simulink model "LinLongNormal_Aquila_ClawsGainSchedule_Discrete"  (Simulink 8.9)
settings: Solver=VariableStepAuto  StartTime=0.0  StopTime=50  RelTol=1e-3  EnableMultiTasking=on
PreLoadFcn:
  | AquilaDiscreteClawsParameters_GS
  | AquilaDiscreteModelParameters
model workspace: external: MAT-File (data not in the file)
undefined symbols (not defined in the file): AP_AltLoop_AltCmdLPFDenTau, AP_AltLoop_Kd0, AP_AltLoop_Ki0, AP_AltLoop_Ki_WindupMaxLim, AP_AltLoop_Ki_WindupMinLim, AP_AltLoop_Kp0, AP_ClimbRate_LPFDenTau, AP_ClimbRateLoop_ClimbRateCmdLPFDenTau, AP_ClimbRateLoop_Ki0, AP_ClimbRateLoop_Kp0, AP_ClimbRateLoop_LLFiltDenCoe0, AP_ClimbRateLoop_LLFiltNumCoe0, AP_ClimbRateLoop_MaxPitchCmdrad, AP_ClimbRateLoop_MinPitchCmdrad, AP_GndTrkLoop_CmdLPFDenTau, AP_GndTrkLoop_Kd0, AP_GndTrkLoop_Kp0, AP_GndTrkLoop_phiCmdMaxLimDeg, AP_GndTrkLoop_phiCmdMinLimDeg, AP_GndTrkLoop_phiRateCmdMaxLimDps, AP_GndTrkLoop_phiRateCmdMinLimDps, AP_PitchLoop_DerivLPFDenTau, AP_PitchLoop_Kd, AP_PitchLoop_Kff, AP_PitchLoop_Ki0, AP_PitchLoop_Kp0, AP_PitchLoop_Kq0, AP_PitchLoop_Notch1BWfactor, AP_PitchLoop_Notch1CosFreqNorm, AP_PitchLoop_qFdbkLFLLFiltDenCoe0, AP_PitchLoop_qFdbkLFLLFiltNumCoe0, AP_PitchLoop_qFdbkLLFiltDenCoe0, AP_PitchLoop_qFdbkLLFiltNumCoe0, AP_PitchLoop_thetaCmdLPFDenTau, AP_PitchLoop_wn_ElvRollOff, AP_PitchLoop_zeta_ElvRollOff, AP_PwrLoop_ClimbRateCmdLPFDenTau, AP_PwrLoop_Ki0, AP_PwrLoop_Kp0, AP_PwrLoop_Kvadv0, AP_PwrLoop_LLFiltDenCoe0, AP_PwrLoop_LLFiltNumCoe0, AP_PwrLoop_MaxThrCmdNorm, AP_PwrLoop_MinThrCmdNorm, AP_PwrLoop_wn_ThrRollOff, AP_PwrLoop_zeta_ThrRollOff, AP_RollLoop_ailCmdMaxLim, AP_RollLoop_ailCmdMinLim, AP_RollLoop_AilWindupMaxLim, AP_RollLoop_AilWindupMinLim, AP_RollLoop_Ki0, AP_RollLoop_Kp0, AP_RollLoop_KrollrateAdv0, AP_RollLoop_Notch1BWfactor, AP_RollLoop_Notch1CosFreqNorm, AP_RollLoop_pFdbkLFLLFiltDenCoe0, AP_RollLoop_pFdbkLFLLFiltNumCoe0, AP_RollLoop_pFdbkLLFiltDenCoe0, AP_RollLoop_pFdbkLLFiltNumCoe0, AP_RollLoop_phiErrLPFDenTau ... (+41)
libraries: discretizing x16, aerolibconvert2 x12, simulink x8
(part 2 of 2)

== system LinLongNormal_Aquila_ClawsGainSchedule_Discrete/Lateral_Directional_Control_Laws/RollLoop/Notch Filter 1 ==
  note: One of ways to implement it for the scheduling of the AP_RollLoop_Notch1CosFreqNorm across the flight envelop
  note: 2nd order IIR Notch filter
  u : Inport
  AP_RollLoop_Notch1BWfactor : Gain  Gain=AP_RollLoop_Notch1BWfactor
  AP_RollLoop_Notch1BWfactor1 : Gain  Gain=AP_RollLoop_Notch1BWfactor
  AP_RollLoop_Notch1BWfactor2 : Gain  Gain=AP_RollLoop_Notch1BWfactor
  AP_RollLoop_Notch1CosFreqNorm : Gain  Gain=AP_RollLoop_Notch1CosFreqNorm
  AP_RollLoop_Notch1CosFreqNorm1 : Gain  Gain=AP_RollLoop_Notch1CosFreqNorm
  Delay : Delay  DelayLength=1  InitialCondition=0  SampleTime=Ts
  Delay1 : Delay  DelayLength=1  InitialCondition=0  SampleTime=Ts
  Delay2 : Delay  InitialCondition=0  SampleTime=Ts
  Delay3 : Delay  InitialCondition=0  SampleTime=Ts
  Gain1 : Gain  Gain=-2
  Gain2 : Gain  Gain=0.4697
  Gain4 : Gain  Gain=2
  Gain5 : Gain  Gain=-1
  Sum : Sum  Inputs=|++
  Sum1 : Sum  Inputs=|++
  Sum2 : Sum  Inputs=|++
  Sum3 : Sum  Inputs=+++||
  y : Outport
  wires:
  Sum/1 -> Gain2/1
  AP_RollLoop_Notch1BWfactor/1 -> Sum/1
  AP_RollLoop_Notch1CosFreqNorm/1 -> Sum3/2
  u/1 -> Delay/1, Sum3/1, Delay2/1
  Sum1/1 -> y/1, Delay1/1, Delay3/1
  AP_RollLoop_Notch1BWfactor2/1 -> Gain5/1
  Delay3/1 -> AP_RollLoop_Notch1BWfactor2/1
  Gain1/1 -> AP_RollLoop_Notch1CosFreqNorm/1
  Delay1/1 -> AP_RollLoop_Notch1CosFreqNorm1/1
  Delay2/1 -> Sum3/3
  Delay/1 -> Gain1/1
  AP_RollLoop_Notch1CosFreqNorm1/1 -> Gain4/1
  Sum3/1 -> Sum/2, AP_RollLoop_Notch1BWfactor/1
  Gain2/1 -> Sum1/1
  Gain4/1 -> Sum2/2
  Gain5/1 -> Sum2/1
  AP_RollLoop_Notch1BWfactor1/1 -> Sum1/2
  Sum2/1 -> AP_RollLoop_Notch1BWfactor1/1

== system LinLongNormal_Aquila_ClawsGainSchedule_Discrete/Lateral_Directional_Control_Laws/RollLoop/Subsystem ==
  note: Return to the previous filter implementation for the opt script
  u : Inport
  pres_alt_m : Inport  Port=2
  DynPres : Inport  Port=3
  AP_RollLoop_pFdbkLLFiltDenCoe : Interpolation_n-D  Table=AP_RollLoop_pFdbkLLFiltDenCoe0  ExtrapMethod=Clip  InternalRulePriority=Speed
  AP_RollLoop_pFdbkLLFiltNumCoe : Interpolation_n-D  Table=AP_RollLoop_pFdbkLLFiltNumCoe0  ExtrapMethod=Clip  InternalRulePriority=Speed
  Delay : Delay  DelayLength=1  InitialCondition=0  SampleTime=Ts
  Prelookup1 : PreLookup  BreakpointsData=0:1500:12000  ExtrapMethod=Linear
  Prelookup2 : PreLookup  BreakpointsData=45:15:150  ExtrapMethod=Linear
  Product1 : Product
  Product2 : Product
  Sum : Sum  Inputs=|++
  Sum1 : Sum  Inputs=+|-
  y : Outport
  wires:
  DynPres/1 -> Prelookup2/1
  AP_RollLoop_pFdbkLLFiltNumCoe/1 -> Product1/2
  AP_RollLoop_pFdbkLLFiltDenCoe/1 -> Product2/2
  pres_alt_m/1 -> Prelookup1/1
  Prelookup1/1 -> AP_RollLoop_pFdbkLLFiltDenCoe/1, AP_RollLoop_pFdbkLLFiltNumCoe/1
  Prelookup1/2 -> AP_RollLoop_pFdbkLLFiltDenCoe/2, AP_RollLoop_pFdbkLLFiltNumCoe/2
  Prelookup2/1 -> AP_RollLoop_pFdbkLLFiltNumCoe/3, AP_RollLoop_pFdbkLLFiltDenCoe/3
  Prelookup2/2 -> AP_RollLoop_pFdbkLLFiltNumCoe/4, AP_RollLoop_pFdbkLLFiltDenCoe/4
  Sum/1 -> y/1, Product2/1
  u/1 -> Sum/1, Product1/1
  Sum1/1 -> Delay/1
  Product1/1 -> Sum1/1
  Delay/1 -> Sum/2
  Product2/1 -> Sum1/2

== system LinLongNormal_Aquila_ClawsGainSchedule_Discrete/Lateral_Directional_Control_Laws/RollLoop/Subsystem3 ==
  u : Inport
  AP_RollLoop_rollAdvLLFiltDenCoe : Gain  Gain=AP_RollLoop_rollAdvLLFiltDenCoe
  AP_RollLoop_rollAdvLLFiltNumCoe : Gain  Gain=AP_RollLoop_rollAdvLLFiltNumCoe
  Delay : Delay  DelayLength=1  InitialCondition=0  SampleTime=Ts
  Delay1 : Delay  DelayLength=1  InitialCondition=0  SampleTime=Ts
  Sum3 : Sum  Inputs=+|+|-
  y : Outport
  wires:
  AP_RollLoop_rollAdvLLFiltDenCoe/1 -> Sum3/3
  u/1 -> AP_RollLoop_rollAdvLLFiltNumCoe/1, Sum3/1
  Delay1/1 -> AP_RollLoop_rollAdvLLFiltDenCoe/1
  AP_RollLoop_rollAdvLLFiltNumCoe/1 -> Delay/1
  Delay/1 -> Sum3/2
  Sum3/1 -> y/1, Delay1/1

== system LinLongNormal_Aquila_ClawsGainSchedule_Discrete/Lateral_Directional_Control_Laws/RollLoop/Subsystem4 ==
  u : Inport
  pres_alt_m : Inport  Port=2
  DynPres : Inport  Port=3
  AP_RollLoop_pFdbkLFLLFiltDenCoe : Interpolation_n-D  Table=AP_RollLoop_pFdbkLFLLFiltDenCoe0  ExtrapMethod=Clip  InternalRulePriority=Speed
  AP_RollLoop_pFdbkLFLLFiltNumCoe : Interpolation_n-D  Table=AP_RollLoop_pFdbkLFLLFiltNumCoe0  ExtrapMethod=Clip  InternalRulePriority=Speed
  Delay : Delay  DelayLength=1  InitialCondition=0  SampleTime=Ts
  Prelookup1 : PreLookup  BreakpointsData=0:1500:12000  ExtrapMethod=Linear
  Prelookup2 : PreLookup  BreakpointsData=45:15:150  ExtrapMethod=Linear
  Product1 : Product
  Product2 : Product
  Sum : Sum  Inputs=|++
  Sum1 : Sum  Inputs=+|-
  y : Outport
  wires:
  DynPres/1 -> Prelookup2/1
  AP_RollLoop_pFdbkLFLLFiltNumCoe/1 -> Product1/2
  AP_RollLoop_pFdbkLFLLFiltDenCoe/1 -> Product2/2
  pres_alt_m/1 -> Prelookup1/1
  Prelookup1/1 -> AP_RollLoop_pFdbkLFLLFiltDenCoe/1, AP_RollLoop_pFdbkLFLLFiltNumCoe/1
  Prelookup1/2 -> AP_RollLoop_pFdbkLFLLFiltDenCoe/2, AP_RollLoop_pFdbkLFLLFiltNumCoe/2
  Prelookup2/1 -> AP_RollLoop_pFdbkLFLLFiltNumCoe/3, AP_RollLoop_pFdbkLFLLFiltDenCoe/3
  Prelookup2/2 -> AP_RollLoop_pFdbkLFLLFiltNumCoe/4, AP_RollLoop_pFdbkLFLLFiltDenCoe/4
  Sum/1 -> y/1, Product2/1
  u/1 -> Sum/1, Product1/1
  Sum1/1 -> Delay/1
  Product1/1 -> Sum1/1
  Delay/1 -> Sum/2
  Product2/1 -> Sum1/2

== system LinLongNormal_Aquila_ClawsGainSchedule_Discrete/Lateral_Directional_Control_Laws/YawLoop/Subsystem1 ==
  u : Inport
  pres_alt_m : Inport  Port=2
  DynPres : Inport  Port=3
  AP_YawRateLoop_LLFiltDenCoe : Interpolation_n-D  Table=AP_YawRateLoop_LLFiltDenCoe0  ExtrapMethod=Clip  InternalRulePriority=Speed
  AP_YawRateLoop_LLFiltNumCoe : Interpolation_n-D  Table=AP_YawRateLoop_LLFiltNumCoe0  ExtrapMethod=Clip  InternalRulePriority=Speed
  Delay : Delay  DelayLength=1  InitialCondition=0  SampleTime=Ts
  Prelookup1 : PreLookup  BreakpointsData=0:1500:12000  ExtrapMethod=Linear
  Prelookup2 : PreLookup  BreakpointsData=45:15:150  ExtrapMethod=Linear
  Product1 : Product
  Product2 : Product
  Sum : Sum  Inputs=|++
  Sum1 : Sum  Inputs=+|-
  y : Outport
  wires:
  DynPres/1 -> Prelookup2/1
  AP_YawRateLoop_LLFiltNumCoe/1 -> Product1/2
  AP_YawRateLoop_LLFiltDenCoe/1 -> Product2/2
  pres_alt_m/1 -> Prelookup1/1
  Prelookup1/1 -> AP_YawRateLoop_LLFiltDenCoe/1, AP_YawRateLoop_LLFiltNumCoe/1
  Prelookup1/2 -> AP_YawRateLoop_LLFiltDenCoe/2, AP_YawRateLoop_LLFiltNumCoe/2
  Prelookup2/1 -> AP_YawRateLoop_LLFiltNumCoe/3, AP_YawRateLoop_LLFiltDenCoe/3
  Prelookup2/2 -> AP_YawRateLoop_LLFiltNumCoe/4, AP_YawRateLoop_LLFiltDenCoe/4
  Sum/1 -> y/1, Product2/1
  u/1 -> Sum/1, Product1/1
  Sum1/1 -> Delay/1
  Product1/1 -> Sum1/1
  Delay/1 -> Sum/2
  Product2/1 -> Sum1/2

== system LinLongNormal_Aquila_ClawsGainSchedule_Discrete/Longitudinal_Control_Laws/ClimbRateLoop/Subsystem1 ==
  pres_alt_m : Inport
  DynPres : Inport  Port=2
  u : Inport  Port=3
  AP_ClimbRateLoop_LLFiltDenCoe : Interpolation_n-D  Table=AP_ClimbRateLoop_LLFiltDenCoe0  ExtrapMethod=Clip  InternalRulePriority=Speed
  AP_ClimbRateLoop_LLFiltNumCoe : Interpolation_n-D  Table=AP_ClimbRateLoop_LLFiltNumCoe0  ExtrapMethod=Clip  InternalRulePriority=Speed
  Delay : Delay  DelayLength=1  InitialCondition=0  SampleTime=Ts
  Delay1 : Delay  DelayLength=1  InitialCondition=0  SampleTime=Ts
  Prelookup1 : PreLookup  BreakpointsData=0:1500:12000  ExtrapMethod=Linear
  Prelookup2 : PreLookup  BreakpointsData=45:15:150  ExtrapMethod=Linear
  Product1 : Product
  Product2 : Product
  Sum3 : Sum  Inputs=+|+|-
  y : Outport
  wires:
  Product2/1 -> Sum3/3
  u/1 -> Sum3/1, Delay/1
  Delay1/1 -> Product2/1
  Product1/1 -> Sum3/2
  Sum3/1 -> y/1, Delay1/1
  DynPres/1 -> Prelookup2/1
  AP_ClimbRateLoop_LLFiltNumCoe/1 -> Product1/2
  AP_ClimbRateLoop_LLFiltDenCoe/1 -> Product2/2
  pres_alt_m/1 -> Prelookup1/1
  Prelookup1/1 -> AP_ClimbRateLoop_LLFiltDenCoe/1, AP_ClimbRateLoop_LLFiltNumCoe/1
  Prelookup1/2 -> AP_ClimbRateLoop_LLFiltDenCoe/2, AP_ClimbRateLoop_LLFiltNumCoe/2
  Prelookup2/1 -> AP_ClimbRateLoop_LLFiltNumCoe/3, AP_ClimbRateLoop_LLFiltDenCoe/3
  Prelookup2/2 -> AP_ClimbRateLoop_LLFiltNumCoe/4, AP_ClimbRateLoop_LLFiltDenCoe/4
  Delay/1 -> Product1/1

== system LinLongNormal_Aquila_ClawsGainSchedule_Discrete/Longitudinal_Control_Laws/PitchLoop/Notch Filter 1 ==
  note: One of ways to implement it for the scheduling of the AP_PitchLoop_Notch1CosFreqNorm across the flight envelop
  note: 2nd order IIR Notch filter
  u : Inport
  AP_PitchLoop_Notch1BWfactor : Gain  Gain=AP_PitchLoop_Notch1BWfactor
  AP_PitchLoop_Notch1BWfactor1 : Gain  Gain=AP_PitchLoop_Notch1BWfactor
  AP_PitchLoop_Notch1BWfactor2 : Gain  Gain=AP_PitchLoop_Notch1BWfactor
  AP_PitchLoop_Notch1CosFreqNorm : Gain  Gain=AP_PitchLoop_Notch1CosFreqNorm
  AP_PitchLoop_Notch1CosFreqNorm1 : Gain  Gain=AP_PitchLoop_Notch1CosFreqNorm
  Delay : Delay  DelayLength=1  InitialCondition=0  SampleTime=Ts
  Delay1 : Delay  DelayLength=1  InitialCondition=0  SampleTime=Ts
  Delay2 : Delay  InitialCondition=0  SampleTime=Ts
  Delay3 : Delay  InitialCondition=0  SampleTime=Ts
  Gain1 : Gain  Gain=-2
  Gain2 : Gain  Gain=0.4697
  Gain4 : Gain  Gain=2
  Gain5 : Gain  Gain=-1
  Sum : Sum  Inputs=|++
  Sum1 : Sum  Inputs=|++
  Sum2 : Sum  Inputs=|++
  Sum3 : Sum  Inputs=+++||
  y : Outport
  wires:
  Sum/1 -> Gain2/1
  AP_PitchLoop_Notch1BWfactor/1 -> Sum/1
  AP_PitchLoop_Notch1CosFreqNorm/1 -> Sum3/2
  u/1 -> Delay/1, Sum3/1, Delay2/1
  Sum1/1 -> y/1, Delay1/1, Delay3/1
  AP_PitchLoop_Notch1BWfactor2/1 -> Gain5/1
  Delay3/1 -> AP_PitchLoop_Notch1BWfactor2/1
  Gain1/1 -> AP_PitchLoop_Notch1CosFreqNorm/1
  Delay1/1 -> AP_PitchLoop_Notch1CosFreqNorm1/1
  Delay2/1 -> Sum3/3
  Delay/1 -> Gain1/1
  AP_PitchLoop_Notch1CosFreqNorm1/1 -> Gain4/1
  Sum3/1 -> Sum/2, AP_PitchLoop_Notch1BWfactor/1
  Gain2/1 -> Sum1/1
  Gain4/1 -> Sum2/2
  Gain5/1 -> Sum2/1
  AP_PitchLoop_Notch1BWfactor1/1 -> Sum1/2
  Sum2/1 -> AP_PitchLoop_Notch1BWfactor1/1

== system LinLongNormal_Aquila_ClawsGainSchedule_Discrete/Longitudinal_Control_Laws/PitchLoop/Subsystem ==
  u : Inport
  pres_alt_m : Inport  Port=2
  DynPres : Inport  Port=3
  AP_PitchLoop_qFdbkLLFiltDenCoe : Interpolation_n-D  Table=AP_PitchLoop_qFdbkLLFiltDenCoe0  InternalRulePriority=Speed
  AP_PitchLoop_qFdbkLLFiltNumCoe : Interpolation_n-D  Table=AP_PitchLoop_qFdbkLLFiltNumCoe0  InternalRulePriority=Speed
  Delay : Delay  DelayLength=1  InitialCondition=0  SampleTime=Ts
  Delay1 : Delay  DelayLength=1  InitialCondition=0  SampleTime=Ts
  Prelookup1 : PreLookup  BreakpointsData=0:1500:12000  ExtrapMethod=Linear
  Prelookup2 : PreLookup  BreakpointsData=45:15:150  ExtrapMethod=Linear
  Product1 : Product
  Product2 : Product
  Sum3 : Sum  Inputs=+|+|-
  y : Outport
  wires:
  Product2/1 -> Sum3/3
  u/1 -> Sum3/1, Delay/1
  Delay1/1 -> Product2/1
  Product1/1 -> Sum3/2
  Sum3/1 -> y/1, Delay1/1
  DynPres/1 -> Prelookup2/1
  AP_PitchLoop_qFdbkLLFiltNumCoe/1 -> Product1/2
  AP_PitchLoop_qFdbkLLFiltDenCoe/1 -> Product2/2
  pres_alt_m/1 -> Prelookup1/1
  Prelookup1/1 -> AP_PitchLoop_qFdbkLLFiltDenCoe/1, AP_PitchLoop_qFdbkLLFiltNumCoe/1
  Prelookup1/2 -> AP_PitchLoop_qFdbkLLFiltDenCoe/2, AP_PitchLoop_qFdbkLLFiltNumCoe/2
  Prelookup2/1 -> AP_PitchLoop_qFdbkLLFiltNumCoe/3, AP_PitchLoop_qFdbkLLFiltDenCoe/3
  Prelookup2/2 -> AP_PitchLoop_qFdbkLLFiltNumCoe/4, AP_PitchLoop_qFdbkLLFiltDenCoe/4
  Delay/1 -> Product1/1

== system LinLongNormal_Aquila_ClawsGainSchedule_Discrete/Longitudinal_Control_Laws/PitchLoop/Subsystem1 ==
  u : Inport
  pres_alt_m : Inport  Port=2
  DynPres : Inport  Port=3
  AP_PitchLoop_qFdbkLFLLFiltDenCoe : Interpolation_n-D  Table=AP_PitchLoop_qFdbkLFLLFiltDenCoe0  InternalRulePriority=Speed
  AP_PitchLoop_qFdbkLFLLFiltNumCoe : Interpolation_n-D  Table=AP_PitchLoop_qFdbkLFLLFiltNumCoe0  InternalRulePriority=Speed
  Delay : Delay  DelayLength=1  InitialCondition=0  SampleTime=Ts
  Delay1 : Delay  DelayLength=1  InitialCondition=0  SampleTime=Ts
  Prelookup1 : PreLookup  BreakpointsData=0:1500:12000  ExtrapMethod=Linear
  Prelookup2 : PreLookup  BreakpointsData=45:15:150  ExtrapMethod=Linear
  Product1 : Product
  Product2 : Product
  Sum3 : Sum  Inputs=+|+|-
  y : Outport
  wires:
  Product2/1 -> Sum3/3
  u/1 -> Sum3/1, Delay/1
  Delay1/1 -> Product2/1
  Product1/1 -> Sum3/2
  Sum3/1 -> y/1, Delay1/1
  DynPres/1 -> Prelookup2/1
  AP_PitchLoop_qFdbkLFLLFiltNumCoe/1 -> Product1/2
  AP_PitchLoop_qFdbkLFLLFiltDenCoe/1 -> Product2/2
  pres_alt_m/1 -> Prelookup1/1
  Prelookup1/1 -> AP_PitchLoop_qFdbkLFLLFiltDenCoe/1, AP_PitchLoop_qFdbkLFLLFiltNumCoe/1
  Prelookup1/2 -> AP_PitchLoop_qFdbkLFLLFiltDenCoe/2, AP_PitchLoop_qFdbkLFLLFiltNumCoe/2
  Prelookup2/1 -> AP_PitchLoop_qFdbkLFLLFiltNumCoe/3, AP_PitchLoop_qFdbkLFLLFiltDenCoe/3
  Prelookup2/2 -> AP_PitchLoop_qFdbkLFLLFiltNumCoe/4, AP_PitchLoop_qFdbkLFLLFiltDenCoe/4
  Delay/1 -> Product1/1

== system LinLongNormal_Aquila_ClawsGainSchedule_Discrete/Longitudinal_Control_Laws/PwrLoop/Subsystem1 ==
  pres_alt_m : Inport
  DynPres : Inport  Port=2
  u : Inport  Port=3
  AP_PwrLoop_LLFiltDenCoe : Interpolation_n-D  Table=AP_PwrLoop_LLFiltDenCoe0  InternalRulePriority=Speed
  AP_PwrLoop_LLFiltNumCoe : Interpolation_n-D  Table=AP_PwrLoop_LLFiltNumCoe0  InternalRulePriority=Speed
  Delay : Delay  DelayLength=1  InitialCondition=0  SampleTime=Ts
  Delay1 : Delay  DelayLength=1  InitialCondition=0  SampleTime=Ts
  Prelookup1 : PreLookup  BreakpointsData=0:1500:12000  ExtrapMethod=Linear
  Prelookup2 : PreLookup  BreakpointsData=45:15:150  ExtrapMethod=Linear
  Product1 : Product
  Product2 : Product
  Sum3 : Sum  Inputs=+|+|-
  y : Outport
  wires:
  Product2/1 -> Sum3/3
  u/1 -> Sum3/1, Delay/1
  Delay1/1 -> Product2/1
  Product1/1 -> Sum3/2
  Sum3/1 -> y/1, Delay1/1
  DynPres/1 -> Prelookup2/1
  AP_PwrLoop_LLFiltNumCoe/1 -> Product1/2
  AP_PwrLoop_LLFiltDenCoe/1 -> Product2/2
  pres_alt_m/1 -> Prelookup1/1
  Prelookup1/1 -> AP_PwrLoop_LLFiltDenCoe/1, AP_PwrLoop_LLFiltNumCoe/1
  Prelookup1/2 -> AP_PwrLoop_LLFiltDenCoe/2, AP_PwrLoop_LLFiltNumCoe/2
  Prelookup2/1 -> AP_PwrLoop_LLFiltNumCoe/3, AP_PwrLoop_LLFiltDenCoe/3
  Prelookup2/2 -> AP_PwrLoop_LLFiltNumCoe/4, AP_PwrLoop_LLFiltDenCoe/4
  Delay/1 -> Product1/1

== system LinLongNormal_Aquila_ClawsGainSchedule_Discrete/Longitudinal_Control_Laws/SpeedLoop/Subsystem ==
  u : Inport
  pres_alt_m : Inport  Port=2
  DynPres : Inport  Port=3
  AP_TASLoop_LLFiltDenCoe : Interpolation_n-D  Table=AP_TASLoop_LLFiltDenCoe0  ExtrapMethod=Clip  InternalRulePriority=Speed
  AP_TASLoop_LLFiltNumCoe : Interpolation_n-D  Table=AP_TASLoop_LLFiltNumCoe0  ExtrapMethod=Clip  InternalRulePriority=Speed
  Delay : Delay  DelayLength=1  InitialCondition=0  SampleTime=Ts
  Delay1 : Delay  DelayLength=1  InitialCondition=0  SampleTime=Ts
  Prelookup1 : PreLookup  BreakpointsData=0:1500:12000  ExtrapMethod=Linear
  Prelookup2 : PreLookup  BreakpointsData=45:15:150  ExtrapMethod=Linear
  Product1 : Product
  Product2 : Product
  Sum3 : Sum  Inputs=+|+|-
  y : Outport
  wires:
  Product2/1 -> Sum3/3
  u/1 -> Sum3/1, Delay/1
  Delay1/1 -> Product2/1
  Product1/1 -> Sum3/2
  Sum3/1 -> y/1, Delay1/1
  DynPres/1 -> Prelookup2/1
  AP_TASLoop_LLFiltNumCoe/1 -> Product1/2
  AP_TASLoop_LLFiltDenCoe/1 -> Product2/2
  pres_alt_m/1 -> Prelookup1/1
  Prelookup1/1 -> AP_TASLoop_LLFiltDenCoe/1, AP_TASLoop_LLFiltNumCoe/1
  Prelookup1/2 -> AP_TASLoop_LLFiltDenCoe/2, AP_TASLoop_LLFiltNumCoe/2
  Prelookup2/1 -> AP_TASLoop_LLFiltNumCoe/3, AP_TASLoop_LLFiltDenCoe/3
  Prelookup2/2 -> AP_TASLoop_LLFiltNumCoe/4, AP_TASLoop_LLFiltDenCoe/4
  Delay/1 -> Product1/1
